simulink model "task3_fin"  (R2020a)
settings: Solver=VariableStepAuto  StartTime=0.0  StopTime=7.0  RelTol=1e-3
values from neighbouring files (symbols this model uses):
  D = [zeros(6); eye(6)]    [task3_script.m]    (also in task3_workspace.mat = [0 0 0 0 0 0 1 0 0 0 0 0 ... (72 elements, 12x6)])
  Kd = 5    [task3_script.m]    (also in task3_workspace.mat)
  Kp = 100    [task3_script.m]    (also in task3_workspace.mat)
  Q = 0.05 * eye(12)    [task3_script.m]    (also in task3_workspace.mat = [5.19109747003 4.48164591787 3.12435266965 3.67324944655 3.6)
  ro = 500    [task3_script.m]
libraries: roblocks x4
settings Model: Creator=root  LastModifiedBy=root

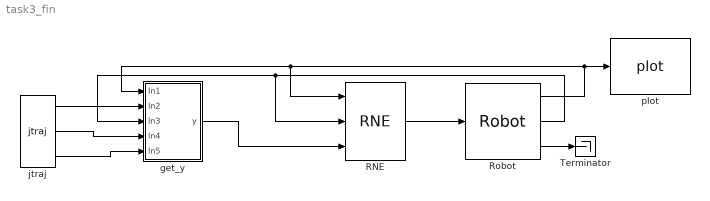
== system task3_fin ==
  RNE : roblocks/Arm/RNE  robot=p560_nf  grav=[0 0 9.81]
  Robot : roblocks/Arm/Robot  robot=p560_nf  q0=[0 0 0 0 0 0]
  Terminator : Terminator
  get_y : Subsystem
  jtraj : roblocks/Toolbox/jtraj  q0=qz  qf=qr  tmax=5.0  ts=0.02
  plot : roblocks/Arm/plot  robot=p560_nf  fps=5  holdplot=on
  wires:
  jtraj/1 -> get_y/2(In2)
  jtraj/2 -> get_y/4(In4)
  Robot/2 -> get_y/3(In3), RNE/2
  RNE/1 -> Robot/1
  get_y/1(y) -> RNE/3
  Robot/1 -> plot/1, get_y/1(In1), RNE/1
  jtraj/3 -> get_y/5(In5)
  Robot/3 -> Terminator/1

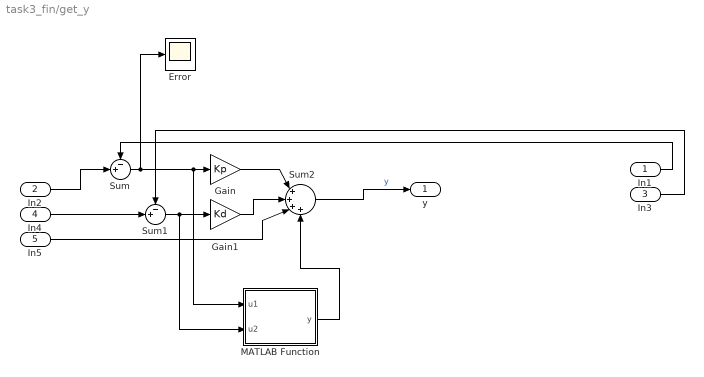
== system task3_fin/get_y ==
  In1 : Inport
  In2 : Inport  Port=2
  In3 : Inport  Port=3
  In4 : Inport  Port=4
  In5 : Inport  Port=5
  Error : Scope
  Gain : Gain  Gain=Kp
  Gain1 : Gain  Gain=Kd
  MATLAB Function : MATLAB Function  TreatAsAtomicUnit=on
  Sum : Sum  Inputs=-+|
  Sum1 : Sum  Inputs=-+|
  Sum2 : Sum  Inputs=|++++
  y : Outport
  wires:
  Sum/1 -> Error/1, MATLAB Function/1(u1), Gain/1
  In1/1 -> Sum/1
  Gain1/1 -> Sum2/2
  Gain/1 -> Sum2/1
  In2/1 -> Sum/2
  Sum2/1 -> y/1  "y"
  Sum1/1 -> MATLAB Function/2(u2), Gain1/1
  In4/1 -> Sum1/2
  In3/1 -> Sum1/1
  In5/1 -> Sum2/3
  MATLAB Function/1(y) -> Sum2/4

== matlab function task3_fin/get_y/MATLAB Function ==
  data: u1 input; y output; u2 input; D parameter; Q parameter; ro parameter
function y = fcn(u1, u2, D, Q, ro)

ksi = [u1;u2];
z = D' * Q * ksi;
z_m = norm(z);

if z_m <= 0.001
    z_m = 0.001;
end

w = ro * (z./z_m);

y = w;
